simulink model "gm_test_ip"  (R2024a)
settings: Solver=FixedStepDiscrete  StartTime=0.0  StopTime=inf  RelTol=1e-3
libraries: hdlsllib x2, simulink x2
settings Model: Creator=versal  LastModifiedBy=versal
settings OptimizationCC: BlockReduction=off  ConditionallyExecuteInputs=off  DefaultParameterBehavior=Inlined  InheritOutputTypeSmallerThanSingle=on
settings DebuggingCC: ArtificialAlgebraicLoopMsg=error  InheritedTsInSrcMsg=none  SingleTaskRateTransMsg=error
settings HardwareCC: ProdBitPerPointer=32  ProdBitPerSizeT=32  ProdBitPerPtrDiffT=32  ProdLargestAtomicFloat=None  ProdIntDivRoundTo=Undefined  ProdEndianess=Unspecified  ProdWordSize=32  ProdHWDeviceType=ASIC/FPGA->ASIC/FPGA  TargetBitPerLong=64  TargetBitPerPointer=64  TargetBitPerSizeT=64  TargetBitPerPtrDiffT=64  TargetLongLongMode=on  TargetIntDivRoundTo=Zero  TargetEndianess=LittleEndian  TargetWordSize=64  TargetHWDeviceType=Custom Processor->MATLAB Host Computer  ProdEqTarget=off

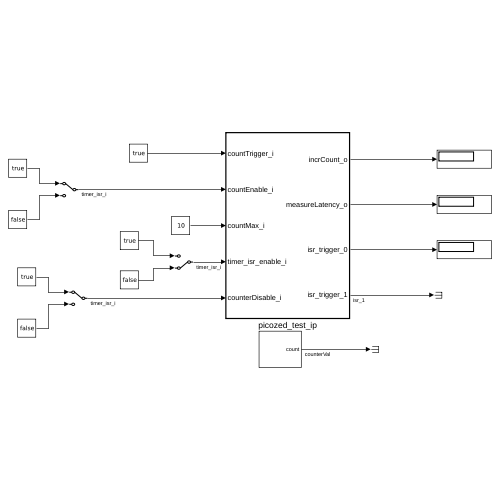
[thumbnail: Simulink's stored preview of the top-level diagram]
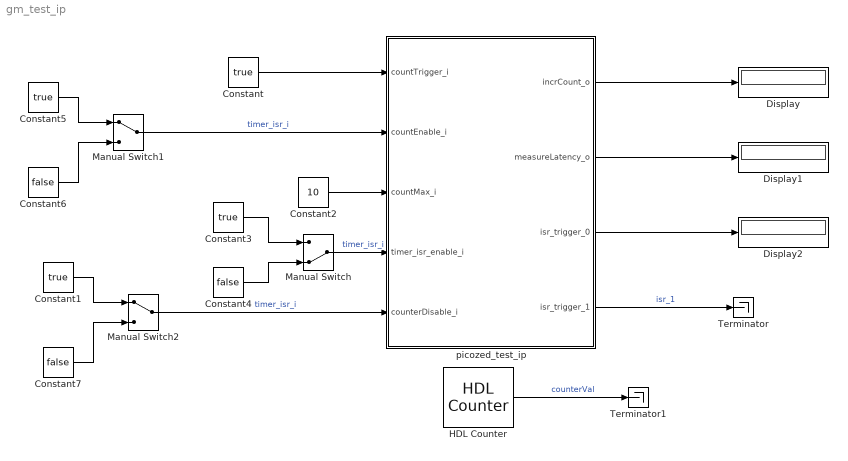
== system gm_test_ip ==
  Constant{,1,3,5} (4 alike) : Constant  Value=true  SampleTime=-1
  Constant2 : Constant  Value=10  OutDataTypeStr=uint32  SampleTime=1
  Constant4 : Constant  Value=false  SampleTime=-1
  Constant6 : Constant  Value=false  SampleTime=-1
  Constant7 : Constant  Value=false  SampleTime=-1
  Display : Display
  Display1 : Display
  Display2 : Display
  HDL Counter : hdlsllib/Sources/HDL Counter  CountType=Free running  CountInit=0  CountStep=1  CountMax=25  CountFromType=Initial value  CountFrom=0  CountResetPort=off  CountLoadPort=off  CountEnbPort=off  CountDirPort=off  CountHitOutputPort=off  CountDataType=Unsigned  CountWordLen=32  CountFracLen=0  CountSampTime=1
  Manual Switch : ManualSwitch  CurrentSetting=0
  Manual Switch1 : ManualSwitch
  Manual Switch2 : ManualSwitch
  Terminator : Terminator
  Terminator1 : Terminator
  picozed_test_ip : Subsystem  TreatAsAtomicUnit=on
  wires:
  Manual Switch2/1 -> picozed_test_ip/5(counterDisable_i)  "timer_isr_i"
  Constant1/1 -> Manual Switch2/1
  Constant7/1 -> Manual Switch2/2
  Manual Switch1/1 -> picozed_test_ip/2(countEnable_i)  "timer_isr_i"
  Constant6/1 -> Manual Switch1/2
  Constant5/1 -> Manual Switch1/1
  Constant4/1 -> Manual Switch/2
  Constant3/1 -> Manual Switch/1
  Manual Switch/1 -> picozed_test_ip/4(timer_isr_enable_i)  "timer_isr_i"
  Constant2/1 -> picozed_test_ip/3(countMax_i)
  HDL Counter/1 -> Terminator1/1  "counterVal"
  picozed_test_ip/4(isr_trigger_1) -> Terminator/1  "isr_1"
  picozed_test_ip/2(measureLatency_o) -> Display1/1
  picozed_test_ip/3(isr_trigger_0) -> Display2/1
  picozed_test_ip/1(incrCount_o) -> Display/1
  Constant/1 -> picozed_test_ip/1(countTrigger_i)

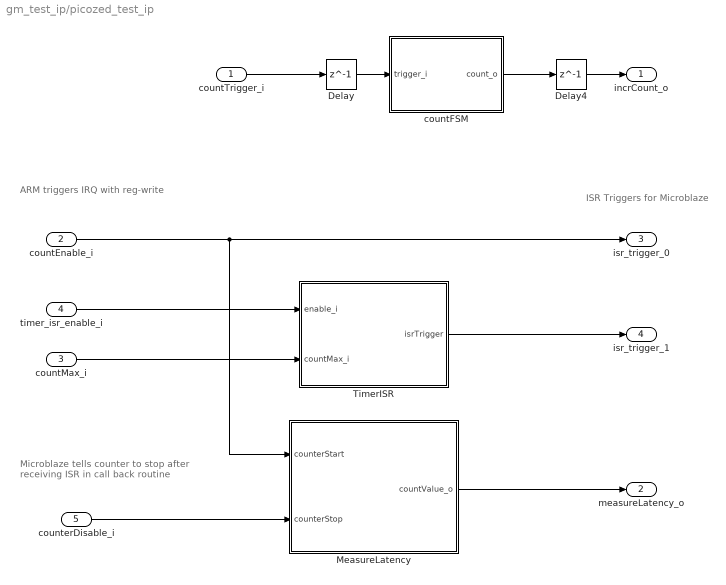
== system gm_test_ip/picozed_test_ip ==
  note: ISR Triggers for Microblaze
  note: ARM triggers IRQ with reg-write
  note: Microblaze tells counter
      | to stop after receiving ISR
      | in call back routine
  countTrigger_i : Inport
  countEnable_i : Inport  Port=2
  countMax_i : Inport  Port=3
  timer_isr_enable_i : Inport  Port=4
  counterDisable_i : Inport  Port=5
  Delay : Delay  DelayLength=1  InitialCondition=0  UseCircularBuffer=on
  Delay4 : Delay  DelayLength=1  InitialCondition=0  UseCircularBuffer=on
  MeasureLatency : Subsystem
  TimerISR : MATLAB Function  TreatAsAtomicUnit=on
  countFSM : MATLAB Function  TreatAsAtomicUnit=on
  incrCount_o : Outport
  measureLatency_o : Outport  Port=2
  isr_trigger_0 : Outport  Port=3
  isr_trigger_1 : Outport  Port=4
  wires:
  counterDisable_i/1 -> MeasureLatency/2(counterStop)
  TimerISR/1(isrTrigger) -> isr_trigger_1/1
  timer_isr_enable_i/1 -> TimerISR/1(enable_i)
  countMax_i/1 -> TimerISR/2(countMax_i)
  Delay4/1 -> incrCount_o/1
  countEnable_i/1 -> MeasureLatency/1(counterStart), isr_trigger_0/1
  MeasureLatency/1(countValue_o) -> measureLatency_o/1
  countFSM/1(count_o) -> Delay4/1
  Delay/1 -> countFSM/1(trigger_i)
  countTrigger_i/1 -> Delay/1

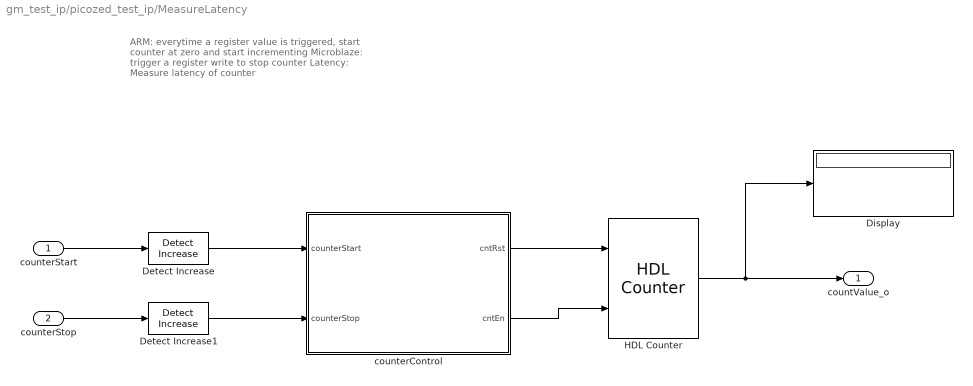
== system gm_test_ip/picozed_test_ip/MeasureLatency ==
  note: ARM: everytime a register value is triggered,
      | start counter at zero and start incrementing
      |
      | Microblaze: trigger a register write to stop counter
      |
      | Latency: Measure latency of counter
  counterStart : Inport
  counterStop : Inport  Port=2
  Detect Increase : simulink/Logic and Bit Operations/Detect Increase  vinit=0.0  OutDataTypeStr=boolean
  Detect Increase1 : simulink/Logic and Bit Operations/Detect Increase  vinit=0.0  OutDataTypeStr=boolean
  Display : Display
  HDL Counter : hdlsllib/Sources/HDL Counter  CountType=Free running  CountInit=0  CountStep=1  CountMax=25  CountFromType=Initial value  CountFrom=0  CountResetPort=on  CountLoadPort=off  CountEnbPort=on  CountDirPort=off  CountHitOutputPort=off  CountDataType=Unsigned  CountWordLen=32  CountFracLen=0  CountSampTime=1
  counterControl : MATLAB Function  TreatAsAtomicUnit=on
  countValue_o : Outport
  wires:
  HDL Counter/1 -> countValue_o/1, Display/1
  counterControl/2(cntEn) -> HDL Counter/2
  counterControl/1(cntRst) -> HDL Counter/1
  Detect Increase/1 -> counterControl/1(counterStart)
  Detect Increase1/1 -> counterControl/2(counterStop)
  counterStop/1 -> Detect Increase1/1
  counterStart/1 -> Detect Increase/1

== matlab function gm_test_ip/picozed_test_ip/countFSM ==
  settings: fimath=fimath('OverflowAction','Wrap')
  data: trigger_i input; count_o output
function count_o = countCtrl(trigger_i)
persistent trigger_reg countValue

if isempty(trigger_reg)
    trigger_reg = false;
    countValue = uint32(0);
end

if (trigger_i == true && trigger_reg == false) % new register poke
    countValue(:) = countValue + 1;
end

count_o = countValue;
trigger_reg = trigger_i;

== matlab function gm_test_ip/picozed_test_ip/MeasureLatency/counterControl ==
  data: cntRst output; counterStart input; counterStop input; cntEn output
function [cntRst,cntEn] = counterControlFcn(counterStart, counterStop)
% Evaluate pulses coming in from counterStart and counterStop
persistent counterState

S_WAIT_FOR_START = fi(0,0,2,0);
S_COUNT_ACTIVE = fi(1,0,2,0);
S_COUNT_STOP = fi(2,0,2,0);

if isempty(counterState)
    counterState = S_WAIT_FOR_START;
end

cntRst = false;
cntEn = false;

switch(counterState)
    case(S_WAIT_FOR_START)
        if counterStart % received pulse to start latency measurement
            counterState(:) = S_COUNT_ACTIVE;
            cntRst  = true;  % reset the counter value before we start counter
        end
    case(S_COUNT_ACTIVE)
        if counterStop % received pulse to stop counting
            counterState(:) = S_WAIT_FOR_START;
        else
            cntEn = true;
        end    
    otherwise
        counterState(:) = S_WAIT_FOR_START;
end



end

== matlab function gm_test_ip/picozed_test_ip/TimerISR ==
  settings: fimath=fimath('OverflowAction','Wrap')
  data: enable_i input; isrTrigger output; countMax_i input
function isrTrigger = timerISR_fcn(enable_i, countMax_i)
persistent countMax_reg timerState counterTick
% If the clock rate is 100 MHz,
% Make default timer 100e6, or, 1 second interrupt timer

%%%
% S_ENABLE_WAIT
% S_COUNTING
% S_MAX_VALUE

S_ENABLE_WAIT = fi(0,0,2,0);
S_COUNTING    = fi(1,0,2,0);
S_MAX_VALUE   = fi(2,0,2,0);
isrTrigger = false;

DEFAULT_TIMER = 100e6;
if isempty(countMax_reg)
    countMax_reg = uint32(DEFAULT_TIMER);
    timerState = S_ENABLE_WAIT;
    counterTick = uint32(0);
end

switch(timerState)
    case(S_ENABLE_WAIT)
        if (countMax_i ~= 0)
            countMax_reg = countMax_i;
        end
        if enable_i
            timerState(:) = S_COUNTING;
        end
    case(S_COUNTING)
        if counterTick >= (countMax_reg - 2) % count when we're one away
            timerState(:) = S_MAX_VALUE;
        end
        counterTick(:) = counterTick + 1;

    case(S_MAX_VALUE)
        % Reached max value, trigger ISR
        counterTick(:) = 0;
        isrTrigger = true;

        if (countMax_i ~= 0)
            countMax_reg = countMax_i;
        end

        if enable_i == false
            timerState(:) = S_ENABLE_WAIT;
        else
            timerState(:) = S_COUNTING;
        end

end
